simulink model "simQuadrotor"  (R2014b)
settings: Solver=ode45  StartTime=0.0  StopTime=tof  FixedStep=dt  MaxStep=dtmax  RelTol=1e-3
values from neighbouring files (symbols this model uses):
  a = (IzzT - IxxT)./ IxxT    [quadrotor.m]
  alpha = 1    [quadrotor.m]
  Aq = -20    [quadrotor.m]
  Ar = -10*eye(2)    [quadrotor.m]
  Arm = [-20 0 ; 0 -5]    [quadrotor.m]
  As = -50*eye(3)    [quadrotor.m]
  attitudeControlFlag = 4    [quadrotor.m]
  Bq = 1    [quadrotor.m]
  Br = [1 0]    [quadrotor.m]
  Dhat0 = zeros(3,1)    [quadrotor.m]
  Dlimit = 2.5    [quadrotor.m]
  DSecondLimit = 2    [quadrotor.m]
  dtFc = 10e-3    (= 0.01)    [quadrotor.m]
  epsilon = 0.1    [quadrotor.m]
  epsilontheta = 0.1    [quadrotor.m]
  euler0 = [0 0 0]'*pi/180    [quadrotor.m]
  Eulerc_ftc = [0 0 0]'    [quadrotor.m]
  faultyPropellerVec = double(not(faultyPropellerVec))    [quadrotor.m]
  FDstart = 3    [quadrotor.m]
  flims = [0.2*0 3.8*2.5]    [quadrotor.m]
  ftc_f2 = 0.1*2    (= 0.2)    [quadrotor.m]
  g = 9.81    [quadrotor.m]
  GammaW = 10000    [quadrotor.m]
  IxxB = IxxT - 4*IxxP    (= 0.0027)    [quadrotor.m]
  IxxT = 2.7e-3    (= 0.0027)    [quadrotor.m]
  IyyB = IyyT - 4*IyyP    (= 0.0027)    [quadrotor.m]
  IyyT = IxxT    (= 0.0027)    [quadrotor.m]
  IzzB = IzzT - 4*IzzP    (= 0.00514)    [quadrotor.m]
  IzzP = 1.5e-5    (= 1.5e-05)    [quadrotor.m]
  IzzT = 5.2e-3    (= 0.0052)    [quadrotor.m]
  Kdxx = 0.7e-4/10    (= 7e-06)    [quadrotor.m]
  Kdzz = 1.4e-4    (= 0.00014)    [quadrotor.m]
  Kf = 6.41e-6    (= 6.41e-06)    [quadrotor.m]
  Kp = 2*0.75*diag([1 1 1])    [quadrotor.m]
  Kp4 = 0.05    [quadrotor.m]
  Ktau = 1.72e-2    (= 0.0172)    [quadrotor.m]
  Kv = 0*0.005*diag([1 1 1])    [quadrotor.m]
  Kv4 = 0.02    [quadrotor.m]
  l = 0.17    [quadrotor.m]
  m = 0.5    [quadrotor.m]
  nc_ftc = 1    [quadrotor.m]
  nCheby = 3    [quadrotor.m]
  pqr0 = [0 0 0]'*pi/180    [quadrotor.m]
  Ps = lyap(As',Q)    [quadrotor.m]
  q0 = [euler0 ; pqr0]    [quadrotor.m]
  qp0 = 0    [quadrotor.m]
  sigmaMot = 0.015    [quadrotor.m]
  tfault = 5    [quadrotor.m]
  Vb0 = [0 0 0]'    [quadrotor.m]
  W0 = 0    [quadrotor.m]
  Wbnd = 10    [quadrotor.m]
  Xe0 = [0 0 0]'    [quadrotor.m]
  xhat0 = [pqr0]    [quadrotor.m]
undefined symbols (not defined in the file or in its folder): Intmax, Intmin, magnitude, rmax, rmin
libraries: aerolibutil x38, simulink x11, vrlib x3, dspbuff3 x1
(part 2 of 3)

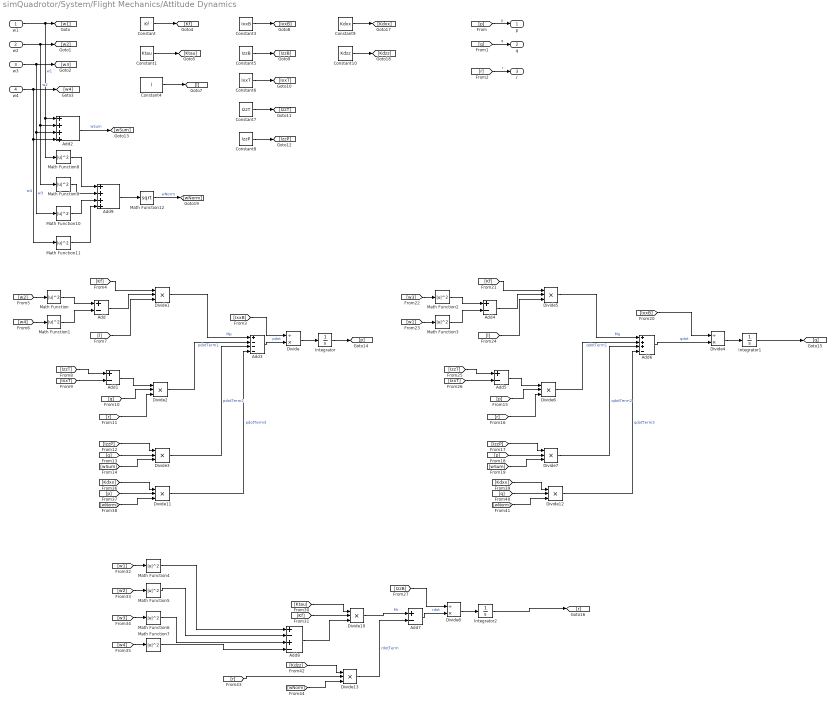
== system simQuadrotor/System/Flight Mechanics/Attitude Dynamics ==
  w1 : Inport
  w2 : Inport  Port=2
  w3 : Inport  Port=3
  w4 : Inport  Port=4
  Add{,1,4..5,7} (5 alike) : Sum  Inputs=+-
  Add2 : Sum  Inputs=++++
  Add3 : Sum  Inputs=+---
  Add6 : Sum  Inputs=+++-
  Add8 : Sum  Inputs=+-+-
  Add9 : Sum  Inputs=++++
  Constant : Constant  Value=Kf
  Constant1 : Constant  Value=Ktau
  Constant10 : Constant  Value=Kdzz
  Constant3 : Constant  Value=IxxB
  Constant4 : Constant  Value=l
  Constant5 : Constant  Value=IzzB
  Constant6 : Constant  Value=IxxT
  Constant7 : Constant  Value=IzzT
  Constant8 : Constant  Value=IzzP
  Constant9 : Constant  Value=Kdxx
  Divide : Product  Inputs=/*
  Divide{1..3,5..7,10..13} (10 alike) : Product  Inputs=***
  Divide4 : Product  Inputs=/*
  Divide8 : Product  Inputs=/*
  Integrator : Integrator  InitialCondition=pqr0(1)
  Integrator1 : Integrator  InitialCondition=pqr0(2)
  Integrator2 : Integrator  InitialCondition=pqr0(3)
  Math Function{,1..11} (12 alike) : Math  Operator=magnitude^2  SaturateOnIntegerOverflow=on
  Math Function12 : Math  Operator=sqrt  SaturateOnIntegerOverflow=on
  p : Outport
  q : Outport  Port=2
  r : Outport  Port=3
  wires:
  w1/1 -> [w1], Add2/1, Math Function8/1  "w1"
  w2/1 -> [w2], Add2/2, Math Function9/1  "w2"
  w3/1 -> [w3], Add2/3, Math Function10/1  "w3"
  w4/1 -> [w4], Add2/4, Math Function11/1  "w4"
  Constant4/1 -> [l]
  Constant1/1 -> [Ktau]
  Constant/1 -> [Kf]
  Constant3/1 -> [IxxB]
  Constant5/1 -> [IzzB]
  Constant6/1 -> [IxxT]
  Constant7/1 -> [IzzT]
  Constant8/1 -> [IzzP]
  [p] -> p/1  "p"
  [q] -> q/1  "q"
  [r] -> r/1  "r"
  Integrator/1 -> [p]
  Divide/1 -> Integrator/1
  [IxxB] -> Divide/1
  [Kf] -> Divide1/1
  [w2] -> Math Function/1
  [w4] -> Math Function1/1
  Math Function/1 -> Add/1
  Math Function1/1 -> Add/2
  Add/1 -> Divide1/2
  [l] -> Divide1/3
  [IzzT] -> Add1/1
  [IxxT] -> Add1/2
  Add1/1 -> Divide2/1
  [q] -> Divide2/2
  [r] -> Divide2/3
  Add2/1 -> [wSum]  "wSum"
  [IzzP] -> Divide3/1
  [q] -> Divide3/2
  [wSum] -> Divide3/3
  Add3/1 -> Divide/2  "pdot"
  Divide1/1 -> Add3/1  "Mp"
  Divide2/1 -> Add3/2  "pdotTerm1"
  Divide3/1 -> Add3/3  "pdotTerm2"
  Integrator1/1 -> [q]
  Divide4/1 -> Integrator1/1
  [IxxB] -> Divide4/1
  [Kf] -> Divide5/1
  [w3] -> Math Function2/1
  [w1] -> Math Function3/1
  Math Function2/1 -> Add4/1
  Math Function3/1 -> Add4/2
  Add4/1 -> Divide5/2
  [l] -> Divide5/3
  [IzzT] -> Add5/1
  [IxxT] -> Add5/2
  Add5/1 -> Divide6/1
  [p] -> Divide6/2
  [r] -> Divide6/3
  [IzzP] -> Divide7/1
  [p] -> Divide7/2
  [wSum] -> Divide7/3
  Add6/1 -> Divide4/2  "qdot"
  Divide5/1 -> Add6/1  "Mq"
  Divide6/1 -> Add6/2  "qdotTerm1"
  Divide7/1 -> Add6/3  "qdotTerm2"
  Integrator2/1 -> [r]
  Divide8/1 -> Integrator2/1
  [IzzB] -> Divide8/1
  Add7/1 -> Divide8/2  "rdot"
  [Ktau] -> Divide10/1
  [Kf] -> Divide10/2
  Add8/1 -> Divide10/3
  [w1] -> Math Function4/1
  [w2] -> Math Function5/1
  Math Function4/1 -> Add8/1
  Math Function5/1 -> Add8/2
  [w3] -> Math Function6/1
  [w4] -> Math Function7/1
  Math Function6/1 -> Add8/3
  Math Function7/1 -> Add8/4
  Constant9/1 -> [Kdxx]
  Constant10/1 -> [Kdzz]
  Math Function8/1 -> Add9/1
  Math Function9/1 -> Add9/2
  Math Function10/1 -> Add9/3
  Math Function11/1 -> Add9/4
  Add9/1 -> Math Function12/1
  Math Function12/1 -> [wNorm]  "wNorm"
  [Kdxx] -> Divide11/1
  [p] -> Divide11/2
  [wNorm] -> Divide11/3
  Divide11/1 -> Add3/4  "pdotTerm3"
  [Kdxx] -> Divide12/1
  [q] -> Divide12/2
  [wNorm] -> Divide12/3
  Divide12/1 -> Add6/4  "qdotTerm3"
  [Kdzz] -> Divide13/1
  [r] -> Divide13/2
  [wNorm] -> Divide13/3
  Divide10/1 -> Add7/1  "Mr"
  Divide13/1 -> Add7/2  "rdotTerm"

== system simQuadrotor/System/Flight Mechanics/DCM E to B ==
  phithetapsi : Inport
  Create 3x3 Matrix : aerolibutil/Create 3x3 Matrix
  Fcn11 : Fcn  Expr=u(5)*u(6)
  Fcn12 : Fcn  Expr=u(3)*u(5)
  Fcn13 : Fcn  Expr=-u(2)
  Fcn21 : Fcn  Expr=u(1)*u(2)*u(6)-u(4)*u(3)
  Fcn22 : Fcn  Expr=u(1)*u(2)*u(3)+u(4)*u(6)
  Fcn23 : Fcn  Expr=u(1)*u(5)
  Fcn31 : Fcn  Expr=u(4)*u(2)*u(6)+u(1)*u(3)
  Fcn32 : Fcn  Expr=u(4)*u(2)*u(3)-u(1)*u(6)
  Fcn33 : Fcn  Expr=u(4)*u(5)
  Mux : Mux  Inputs=2
  sincos : Trigonometry  Operator=sincos
  CB_E : Outport
  wires:
  sincos/1 -> Mux/1
  sincos/2 -> Mux/2
  Mux/1 -> Fcn32/1, Fcn33/1, Fcn31/1, Fcn23/1, Fcn22/1, Fcn11/1, Fcn12/1, Fcn13/1, Fcn21/1
  Fcn11/1 -> Create 3x3 Matrix/1
  Fcn12/1 -> Create 3x3 Matrix/2
  Fcn13/1 -> Create 3x3 Matrix/3
  Fcn21/1 -> Create 3x3 Matrix/4
  Fcn31/1 -> Create 3x3 Matrix/7
  Fcn22/1 -> Create 3x3 Matrix/5
  Fcn23/1 -> Create 3x3 Matrix/6
  Fcn32/1 -> Create 3x3 Matrix/8
  Fcn33/1 -> Create 3x3 Matrix/9
  phithetapsi/1 -> sincos/1  "phithetapsi"
  Create 3x3 Matrix/1 -> CB_E/1  "CB_E"

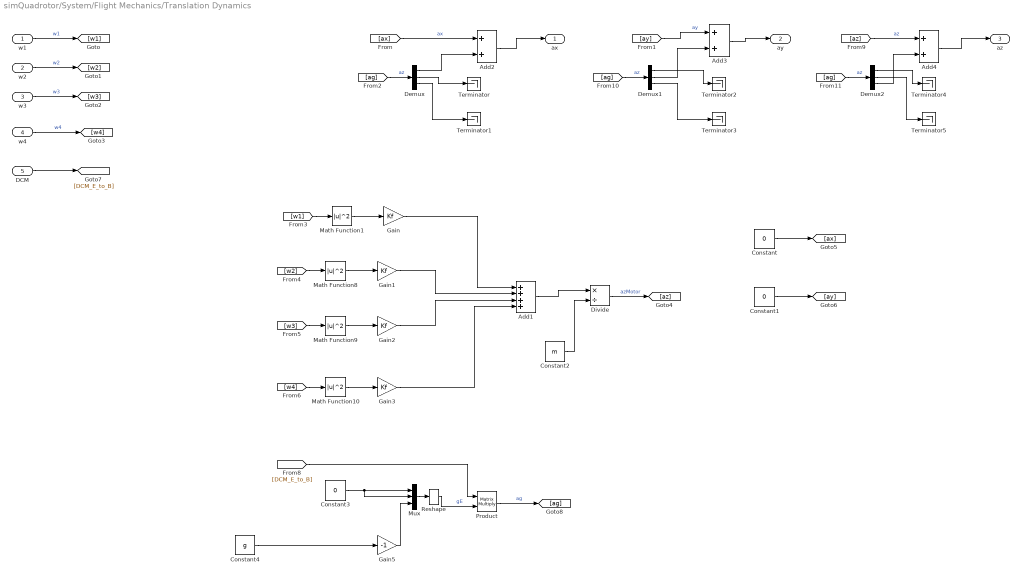
== system simQuadrotor/System/Flight Mechanics/Translation Dynamics ==
  w1 : Inport
  w2 : Inport  Port=2
  w3 : Inport  Port=3
  w4 : Inport  Port=4
  DCM : Inport  Port=5
  Add1 : Sum  Inputs=++++
  Add2 : Sum
  Add3 : Sum
  Add4 : Sum
  Constant : Constant  Value=0
  Constant1 : Constant  Value=0
  Constant2 : Constant  Value=m
  Constant3 : Constant  Value=0
  Constant4 : Constant  Value=g
  Demux : Demux  Outputs=3
  Demux1 : Demux  Outputs=3
  Demux2 : Demux  Outputs=3
  Divide : Product  Inputs=*/
  Gain{,1..3} (4 alike) : Gain  Gain=Kf
  Gain5 : Gain  Gain=-1
  Math Function{1,8..10} (4 alike) : Math  Operator=magnitude^2  SaturateOnIntegerOverflow=on
  Mux : Mux  Inputs=3
  Product : Product  Multiplication=Matrix(*)  RndMeth=Zero
  Reshape : Reshape  OutputDimensionality=Column vector (2-D)
  Terminator{,1..5} (6 alike) : Terminator
  ax : Outport
  ay : Outport  Port=2
  az : Outport  Port=3
  wires:
  w4/1 -> [w4]  "w4"
  w3/1 -> [w3]  "w3"
  w2/1 -> [w2]  "w2"
  w1/1 -> [w1]  "w1"
  [w1] -> Math Function1/1
  Math Function1/1 -> Gain/1
  [w2] -> Math Function8/1
  Math Function8/1 -> Gain1/1
  [w3] -> Math Function9/1
  Math Function9/1 -> Gain2/1
  [w4] -> Math Function10/1
  Math Function10/1 -> Gain3/1
  Gain/1 -> Add1/1
  Gain1/1 -> Add1/2
  Gain2/1 -> Add1/3
  Gain3/1 -> Add1/4
  Constant4/1 -> Gain5/1
  Constant/1 -> [ax]
  Constant1/1 -> [ay]
  Add1/1 -> Divide/1
  Divide/1 -> [az]  "azMotor"
  Constant2/1 -> Divide/2
  DCM/1 -> [DCM_E_to_B]
  [DCM_E_to_B] -> Product/1
  Constant3/1 -> Mux/1, Mux/2
  Gain5/1 -> Mux/3
  Mux/1 -> Reshape/1
  Reshape/1 -> Product/2  "gE"
  Product/1 -> [ag]  "ag"
  [ag] -> Demux/1  "az"
  [ax] -> Add2/1  "ax"
  Add2/1 -> ax/1
  [ay] -> Add3/1  "ay"
  Add3/1 -> ay/1
  [az] -> Add4/1  "az"
  Add4/1 -> az/1
  Demux/1 -> Add2/2
  [ag] -> Demux1/1  "az"
  Demux1/2 -> Add3/2
  [ag] -> Demux2/1  "az"
  Demux2/3 -> Add4/2
  Demux/2 -> Terminator/1
  Demux/3 -> Terminator1/1
  Demux1/1 -> Terminator2/1
  Demux1/3 -> Terminator3/1
  Demux2/1 -> Terminator4/1
  Demux2/2 -> Terminator5/1

== system simQuadrotor/System/Navigation/DCM E to B ==
  phithetapsi : Inport
  Create 3x3 Matrix : aerolibutil/Create 3x3 Matrix
  Fcn11 : Fcn  Expr=u(5)*u(6)
  Fcn12 : Fcn  Expr=u(3)*u(5)
  Fcn13 : Fcn  Expr=-u(2)
  Fcn21 : Fcn  Expr=u(1)*u(2)*u(6)-u(4)*u(3)
  Fcn22 : Fcn  Expr=u(1)*u(2)*u(3)+u(4)*u(6)
  Fcn23 : Fcn  Expr=u(1)*u(5)
  Fcn31 : Fcn  Expr=u(4)*u(2)*u(6)+u(1)*u(3)
  Fcn32 : Fcn  Expr=u(4)*u(2)*u(3)-u(1)*u(6)
  Fcn33 : Fcn  Expr=u(4)*u(5)
  Math Function : Math  Operator=transpose  SaturateOnIntegerOverflow=on
  Mux : Mux  Inputs=2
  Product : Product  Multiplication=Matrix(*)  RndMeth=Zero
  Product1 : Product  Inputs=/  Multiplication=Matrix(*)  RndMeth=Zero
  Terminator : Terminator
  Terminator1 : Terminator
  sincos : Trigonometry  Operator=sincos
  CB_E : Outport
  wires:
  sincos/1 -> Mux/1
  sincos/2 -> Mux/2
  Mux/1 -> Fcn32/1, Fcn33/1, Fcn31/1, Fcn23/1, Fcn22/1, Fcn11/1, Fcn12/1, Fcn13/1, Fcn21/1
  Fcn11/1 -> Create 3x3 Matrix/1
  Fcn12/1 -> Create 3x3 Matrix/2
  Fcn13/1 -> Create 3x3 Matrix/3
  Fcn21/1 -> Create 3x3 Matrix/4
  Fcn31/1 -> Create 3x3 Matrix/7
  Fcn22/1 -> Create 3x3 Matrix/5
  Fcn23/1 -> Create 3x3 Matrix/6
  Fcn32/1 -> Create 3x3 Matrix/8
  Fcn33/1 -> Create 3x3 Matrix/9
  phithetapsi/1 -> sincos/1  "phithetapsi"
  Create 3x3 Matrix/1 -> Math Function/1, CB_E/1, Product/1, Product1/1  "CB_E"
  Math Function/1 -> Product/2  "CB_ET"
  Product1/1 -> Terminator1/1  "CB_E_inv"
  Product/1 -> Terminator/1  "mult"

== system simQuadrotor/Controller/Disturbance Estimator/getDisturbance/Chebyshev Basis Functions ==
  x : Inport
  Chebyshev Polynomail Value Calculation : Subsystem  TreatAsAtomicUnit=on
  Demux : Demux  Outputs=3
  Mux : Mux  Inputs=3
  Reshape1 : Reshape  OutputDimensionality=Column vector (2-D)
  Reshape2 : Reshape  OutputDimensionality=Column vector (2-D)
  Tn : Outport
  wires:
  [Tn] -> Tn/1
  [z] -> Chebyshev Polynomail Value Calculation/1(x)
  Chebyshev Polynomail Value Calculation/1(chebyPol) -> Reshape2/1
  Reshape2/1 -> [Tn]
  x/1 -> [x]
  Mux/1 -> Reshape1/1
  Reshape1/1 -> [z]
  [x] -> Demux/1
  [wB2] -> Mux/2
  [wB3] -> Mux/3
  [wB1] -> Mux/1
  Demux/1 -> [wB1]
  Demux/2 -> [wB2]
  Demux/3 -> [wB3]

== system simQuadrotor/Controller/Disturbance Estimator/getDisturbance/getDhat ==
  psiz : Inport
  es : Inport  Port=2
  Bus Creator : BusCreator  Inputs=3
  Math Function : Math  Operator=transpose  SaturateOnIntegerOverflow=on
  Math Function1 : Math  Operator=transpose  SaturateOnIntegerOverflow=on
  Math Function2 : Math  Operator=transpose  SaturateOnIntegerOverflow=on
  Reshape : Reshape  OutputDimensionality=Column vector (2-D)
  Selector : Selector  NumberOfDimensions=2  InputPortWidth=3  IndexOptions=Select all,Index vector (dialog)  Indices=[1 3],1  OutputSizes=1,1
  Selector1 : Selector  NumberOfDimensions=2  InputPortWidth=3  IndexOptions=Select all,Index vector (dialog)  Indices=[1 3],2  OutputSizes=1,1
  Selector2 : Selector  NumberOfDimensions=2  InputPortWidth=3  IndexOptions=Select all,Index vector (dialog)  Indices=[1 3],3  OutputSizes=1,1
  Terminator1 : Terminator
  Vector Concatenate : Concatenate  NumInputs=3
  adaptiveGain : Subsystem  TreatAsAtomicUnit=on
  getW1 : Subsystem
  getW2 : Subsystem
  getW3 : Subsystem
  Dhat : Outport
  wires:
  es/1 -> [es]  "es"
  adaptiveGain/1(Wintegrand) -> [Wint]  "Wint"
  [Dhat] -> Dhat/1  "Dhat"
  psiz/1 -> [psiz]  "psiz"
  [es] -> adaptiveGain/2(es)
  [psiz] -> adaptiveGain/1(psi(z))
  [psiz] -> getW1/2(psiz)
  Selector/1 -> getW1/1(Wint)
  Vector Concatenate/1 -> Reshape/1
  [psiz] -> getW2/2(psiz)
  Selector1/1 -> getW2/1(Wint)
  Reshape/1 -> [Dhat]
  Bus Creator/1 -> Terminator1/1  "W"
  getW2/2(WTpsi) -> Vector Concatenate/2
  getW1/2(WTpsi) -> Vector Concatenate/1
  getW1/1(W) -> Math Function/1
  getW2/1(W) -> Math Function1/1
  [Wint] -> Selector2/1, Selector1/1, Selector/1
  Math Function/1 -> Bus Creator/1  "W1"
  Math Function1/1 -> Bus Creator/2  "W2"
  Selector2/1 -> getW3/1(Wint)
  [psiz] -> getW3/2(psiz)
  getW3/1(W) -> Math Function2/1
  Math Function2/1 -> Bus Creator/3
  getW3/2(WTpsi) -> Vector Concatenate/3  "W3"

== system simQuadrotor/Controller/FTC Controller/SingleProp Compensation/Motor Force Calculation ==
  fc : Inport
  u : Inport  Port=2
  Add2 : Sum  Inputs=+-
  Add3 : Sum
  Constant1 : Constant  Value=ftc_f2  VectorParams1D=off
  Constant3 : Constant  Value=0  VectorParams1D=off
  Gain1 : Gain  Gain=1/l
  Gain{3..4,9..10} (4 alike) : Gain  Gain=1/2
  Gain2 : Gain  Gain=1/l
  Mux : Mux
  Reshape : Reshape  OutputDimensionality=Column vector (2-D)
  fic : Outport
  wires:
  Gain4/1 -> Add3/1
  Gain3/1 -> Add2/1
  Gain2/1 -> Add3/2
  Gain1/1 -> Add2/2
  Gain10/1 -> Gain2/1
  Gain9/1 -> Gain1/1
  Constant1/1 -> [f2]
  u/1 -> [u]  "u"
  [f3] -> Mux/3
  [f1] -> Mux/1
  [f4] -> Mux/4
  [f2] -> Mux/2
  Constant3/1 -> [f4]
  Reshape/1 -> [fic]  "fic"
  Add3/1 -> [f3]
  [fc] -> Gain4/1
  [u] -> Gain10/1
  Add2/1 -> [f1]
  [fc] -> Gain3/1
  [u] -> Gain9/1
  Mux/1 -> Reshape/1
  [fic] -> fic/1
  fc/1 -> [fc]  "fc"

== system simQuadrotor/Controller/FTC Controller/SingleProp Compensation/PD-control for Reduced Attitude-Bullo ==
  r : Inport
  x : Inport  Port=2
  Add1 : Sum  Inputs=+-
  Constant1 : Constant  Value=0  VectorParams1D=off
  Gain4 : Gain  Gain=-1  Multiplication=Matrix(K*u)
  Gain5 : Gain  Gain=Kp4
  Gain6 : Gain  Gain=Kv4
  Math Function2 : Math  Operator=transpose  SaturateOnIntegerOverflow=on
  Math Function3 : Math  Operator=transpose  SaturateOnIntegerOverflow=on
  Mux : Mux  Inputs=2
  Mux1 : Mux  Inputs=2
  Mux2 : Mux  Inputs=2
  Product2 : Product  Multiplication=Matrix(*)  RndMeth=Zero
  Product3 : Product  Multiplication=Matrix(*)  RndMeth=Zero
  Product4 : Product  RndMeth=Zero
  Reshape{,1..4} (5 alike) : Reshape  OutputDimensionality=Column vector (2-D)
  "[4 5 6]" : Selector  InputPortWidth=6  Indices=4
  "[4 5 6]1" : Selector  InputPortWidth=6  Indices=5
  getRedAttRelatedPars : Subsystem
  Mc : Outport
  wires:
  Reshape4/1 -> [Mc]
  Constant1/1 -> Mux2/2
  Add1/1 -> Mux2/1
  Mux2/1 -> Reshape4/1
  Gain6/1 -> Add1/2  "Kvterm"
  Gain5/1 -> Add1/1  "Kpterm"
  Reshape2/1 -> Gain6/1
  [w2] -> Mux1/2
  [w1] -> Mux1/1
  Mux1/1 -> Reshape2/1
  Product4/1 -> Gain5/1
  Reshape/1 -> Product4/2
  [dist_pi0_q] -> Product4/1
  Mux/1 -> Reshape/1
  [V_Ypi1_V] -> Mux/2
  Gain4/1 -> Mux/1
  [V_Ypi2_V] -> Gain4/1
  [x] -> "[4 5 6]1"/1
  "[4 5 6]1"/1 -> Reshape1/1
  Reshape1/1 -> [w2]  "w2"
  [x] -> "[4 5 6]"/1
  "[4 5 6]"/1 -> Reshape3/1
  Reshape3/1 -> [w1]  "w1"
  Product3/1 -> [V_Ypi1_V]
  [pi1] -> Product3/2
  Math Function3/1 -> Product3/1
  [Yq_pi0] -> Math Function3/1
  Product2/1 -> [V_Ypi2_V]
  [pi2] -> Product2/2
  Math Function2/1 -> Product2/1
  [Yq_pi0] -> Math Function2/1
  getRedAttRelatedPars/4(pi2) -> [pi2]
  getRedAttRelatedPars/3(pi1) -> [pi1]
  getRedAttRelatedPars/1(Yq_pi0) -> [Yq_pi0]
  getRedAttRelatedPars/2(dist_pi0_q) -> [dist_pi0_q]
  [r] -> getRedAttRelatedPars/1(r)
  [x] -> getRedAttRelatedPars/2(x)
  [Mc] -> Mc/1  "Mc"
  x/1 -> [x]  "x"
  r/1 -> [r]  "r"

== system simQuadrotor/Controller/FTC Controller/SingleProp Compensation/Perturbation Calculation ==
  x : Inport
  qc : Inport  Port=2
  Add : Sum  Inputs=+-
  Add1 : Sum
  Add2 : Sum
  Add3 : Sum
  Constant1 : Constant  Value=Br  VectorParams1D=off
  Discrete-Time Integrator : DiscreteIntegrator  IntegratorMethod=Integration: Backward Euler  InitialCondition=qp0  InitialConditionSetting=State (most efficient)  SampleTime=-1  UpperSaturationLimit=rmax  LowerSaturationLimit=rmin
  Gain1 : Gain  Gain=Br'
  Gain2 : Gain  Gain=[0 0 0 0 1 0]'
  Gain3 : Gain  Gain=1/epsilon
  Gain4 : Gain  Gain=alpha
  Gain8 : Gain  Gain=Ar  Multiplication=Matrix(K*u)
  Memory3 : Memory  X0=qp0  InheritSampleTime=on  LinearizeMemory=on  LinearizeAsDelay=on
  Product1 : Product  Multiplication=Matrix(*)
  Reference model : Subsystem  TreatAsAtomicUnit=on
  Reshape2 : Reshape  OutputDimensionality=Column vector (2-D)
  System model : Subsystem  TreatAsAtomicUnit=on
  Terminator : Terminator
  getStates : Subsystem
  qp : Outport
  wires:
  [p2p] -> System model/5(p2p)
  [p1p] -> System model/4(p1p)
  getStates/5(p2p) -> [p2p]
  getStates/4(p1p) -> [p1p]
  [x2] -> Terminator/1
  Product1/1 -> [qp]
  [r] -> Product1/2
  Constant1/1 -> Product1/1
  [x1] -> System model/1(x1)
  getStates/3(w3) -> [w3]
  getStates/2(x2) -> [x2]
  getStates/1(x1) -> [x1]
  x/1 -> [x]  "x"
  [qp] -> qp/1
  System model/1(f1) -> [f1]  "f1"
  [w3] -> System model/2(w3)
  Reshape2/1 -> Memory3/1
  [r] -> Gain8/1
  Discrete-Time Integrator/1 -> Reshape2/1
  Gain3/1 -> Discrete-Time Integrator/1
  Memory3/1 -> [r]  "r"
  Gain8/1 -> Add2/2
  Reference model/1(f1r) -> [f1r]  "f1r"
  [x1] -> Reference model/1(x1)
  Add2/1 -> Gain3/1
  Gain4/1 -> Add2/1
  [f1r] -> Add/2
  [f1] -> Add/1
  Add/1 -> Gain4/1  "r_rhs"
  qc/1 -> [qc]  "qc"
  Add1/1 -> System model/3(r)
  [r] -> Add1/1
  [qc] -> Gain1/1
  Gain1/1 -> Add1/2
  [qc] -> Gain2/1
  [x] -> Add3/1
  Gain2/1 -> Add3/2
  Add3/1 -> getStates/1(x)

== system simQuadrotor/Controller/FTC Controller/SingleProp Compensation/Required Total Thrust ==
  x : Inport
  nc : Inport  Port=2
  Constant : Constant
  Constant1 : Constant  Value=m
  Constant2 : Constant  Value=g
  Product of Elements : Product  Inputs=*
  Product1 : Product  RndMeth=Zero
  Product2 : Product  Inputs=**/  RndMeth=Zero
  Selector : Selector  NumberOfDimensions=2  InputPortWidth=3  IndexOptions=Index vector (dialog),Index vector (dialog)  Indices=[1 2],1  OutputSizes=1,1
  Terminator : Terminator
  Trigonometric Function : Trigonometry  Operator=cos
  fc : Outport
  wires:
  Product1/1 -> Product2/2
  [nc] -> Product2/1
  nc/1 -> [nc]
  Trigonometric Function/1 -> Product of Elements/1
  Product of Elements/1 -> [cosphi_costht]
  Selector/1 -> Trigonometric Function/1
  Product2/1 -> fc/1
  Constant2/1 -> Product1/2
  Constant1/1 -> Product1/1
  x/1 -> Selector/1
  [cosphi_costht] -> Product2/3
  Constant/1 -> Terminator/1

== system simQuadrotor/Controller/FTC Controller/SingleProp Compensation/w3 Controller ==
  x : Inport
  qp : Inport  Port=2
  qc : Inport  Port=3
  Add1 : Sum
  Add2 : Sum  Inputs=++-
  Constant2 : Constant  Value=a  VectorParams1D=off
  Gain1 : Gain  Gain=Aq
  Gain2 : Gain  Gain=IyyT
  Gain3 : Gain  Gain=Bq
  Product1 : Product  Inputs=3  RndMeth=Zero
  Reshape1 : Reshape  OutputDimensionality=Column vector (2-D)
  Reshape3 : Reshape  OutputDimensionality=Column vector (2-D)
  Reshape5 : Reshape  OutputDimensionality=Column vector (2-D)
  "[4 5 6]" : Selector  InputPortWidth=6  Indices=4
  "[4 5 6]1" : Selector  InputPortWidth=6  Indices=6
  "[4 5 6]2" : Selector  InputPortWidth=6  Indices=5
  Mc : Outport
  wires:
  qp/1 -> [qp]  "qp"
  Gain2/1 -> [Mc]
  Add2/1 -> Gain2/1
  [w2] -> Gain1/1
  Reshape5/1 -> [w2]  "w2"
  "[4 5 6]2"/1 -> Reshape5/1
  [x] -> "[4 5 6]2"/1
  Constant2/1 -> Product1/1
  [w3] -> Product1/3
  [w1] -> Product1/2
  qc/1 -> [qc]  "qc"
  x/1 -> [x]  "x"
  [Mc] -> Mc/1  "Mc"
  Reshape3/1 -> [w1]  "w1"
  "[4 5 6]"/1 -> Reshape3/1
  [x] -> "[4 5 6]"/1
  Reshape1/1 -> [w3]  "w3"
  "[4 5 6]1"/1 -> Reshape1/1
  [x] -> "[4 5 6]1"/1
  Add1/1 -> Gain3/1  "qcommand"
  [qp] -> Add1/1
  [qc] -> Add1/2
  Gain3/1 -> Add2/1
  Gain1/1 -> Add2/2
  Product1/1 -> Add2/3

== system simQuadrotor/Controller/Nominal Controller/PD-Attitude Control with wB_IB/get eR ==
  r : Inport
  q : Inport  Port=2
  Add1 : Sum  Inputs=+-
  Add2 : Sum  Inputs=+-
  DCM E to B : Subsystem
  DCM E to B1 : Subsystem
  Product2 : Product  Inputs=/  Multiplication=Matrix(*)  RndMeth=Zero
  Product5 : Product  Inputs=/  Multiplication=Matrix(*)  RndMeth=Zero
  Product6 : Product  Multiplication=Matrix(*)  RndMeth=Zero
  Reshape{1..5} (5 alike) : Reshape  OutputDimensionality=Column vector (2-D)
  Terminator1 : Terminator
  Terminator2 : Terminator
  Terminator3 : Terminator
  "[ 1 2 3]" : Selector  NumberOfDimensions=2  InputPortWidth=3  IndexOptions=Index vector (dialog),Index vector (dialog)  Indices=[1 2 3],1  OutputSizes=1,1
  "[2 3 4]" : Selector  NumberOfDimensions=2  InputPortWidth=3  IndexOptions=Index vector (dialog),Index vector (dialog)  Indices=[2 3 4],1  OutputSizes=1,1
  "[4 5 6]" : Selector  NumberOfDimensions=2  InputPortWidth=3  IndexOptions=Index vector (dialog),Index vector (dialog)  Indices=[4 5 6],1  OutputSizes=1,1
  get Omega(R) RBAC : Subsystem
  get eR : Subsystem
  eR : Outport
  wires:
  [R] -> get eR/2(R)
  get eR/1(eR) -> [eR]  "eR"
  [Rc] -> get eR/1(Rc)
  [R] -> get Omega(R) RBAC/2(R)
  Product5/1 -> [R]
  Product2/1 -> [Rc]
  [q] -> Reshape5/1
  "[ 1 2 3]"/1 -> Reshape2/1
  "[4 5 6]"/1 -> Reshape3/1
  Reshape5/1 -> "[ 1 2 3]"/1, "[4 5 6]"/1
  [Rc] -> Product6/1  "RcTR"
  [wB] -> Product6/2
  [wB] -> Add1/1
  Product6/1 -> Add1/2  "RcTRpqr"
  Add1/1 -> Terminator1/1  "eM"
  [Euler] -> Add2/1
  [Eulerc] -> Add2/2
  Add2/1 -> Terminator2/1  "eEuler"
  get Omega(R) RBAC/1(Omega(R)) -> Terminator3/1  "Omega_R_"
  [Rc] -> get Omega(R) RBAC/1(Rc)
  Reshape1/1 -> [Eulerc]
  "[2 3 4]"/1 -> Reshape1/1
  [r] -> Reshape4/1
  Reshape2/1 -> [Euler]  "Euler"
  Reshape3/1 -> [wB]  "wB"
  Reshape4/1 -> "[2 3 4]"/1
  [Eulerc] -> DCM E to B/1(phithetapsi)
  DCM E to B/1(CB_E) -> Product2/1
  [Euler] -> DCM E to B1/1(phithetapsi)
  DCM E to B1/1(CB_E) -> Product5/1
  [eR] -> eR/1
  r/1 -> [r]  "r"
  q/1 -> [q]  "q"

== system simQuadrotor/Controller/Nominal Controller/PD-control for Attitude/DCM E to B ==
  phithetapsi : Inport
  Create 3x3 Matrix : aerolibutil/Create 3x3 Matrix
  Fcn11 : Fcn  Expr=u(5)*u(6)
  Fcn12 : Fcn  Expr=u(3)*u(5)
  Fcn13 : Fcn  Expr=-u(2)
  Fcn21 : Fcn  Expr=u(1)*u(2)*u(6)-u(4)*u(3)
  Fcn22 : Fcn  Expr=u(1)*u(2)*u(3)+u(4)*u(6)
  Fcn23 : Fcn  Expr=u(1)*u(5)
  Fcn31 : Fcn  Expr=u(4)*u(2)*u(6)+u(1)*u(3)
  Fcn32 : Fcn  Expr=u(4)*u(2)*u(3)-u(1)*u(6)
  Fcn33 : Fcn  Expr=u(4)*u(5)
  Mux : Mux  Inputs=2
  sincos : Trigonometry  Operator=sincos
  CB_E : Outport
  wires:
  Create 3x3 Matrix/1 -> CB_E/1  "CB_E"
  phithetapsi/1 -> sincos/1  "phithetapsi"
  Fcn33/1 -> Create 3x3 Matrix/9
  Fcn32/1 -> Create 3x3 Matrix/8
  Fcn23/1 -> Create 3x3 Matrix/6
  Fcn22/1 -> Create 3x3 Matrix/5
  Fcn31/1 -> Create 3x3 Matrix/7
  Fcn21/1 -> Create 3x3 Matrix/4
  Fcn13/1 -> Create 3x3 Matrix/3
  Fcn12/1 -> Create 3x3 Matrix/2
  Fcn11/1 -> Create 3x3 Matrix/1
  Mux/1 -> Fcn21/1, Fcn13/1, Fcn12/1, Fcn11/1, Fcn22/1, Fcn23/1, Fcn31/1, Fcn33/1, Fcn32/1
  sincos/2 -> Mux/2
  sincos/1 -> Mux/1

== system simQuadrotor/Controller/Nominal Controller/PD-control for Attitude/DCM E to B1 ==
  phithetapsi : Inport
  Create 3x3 Matrix : aerolibutil/Create 3x3 Matrix
  Fcn11 : Fcn  Expr=u(5)*u(6)
  Fcn12 : Fcn  Expr=u(3)*u(5)
  Fcn13 : Fcn  Expr=-u(2)
  Fcn21 : Fcn  Expr=u(1)*u(2)*u(6)-u(4)*u(3)
  Fcn22 : Fcn  Expr=u(1)*u(2)*u(3)+u(4)*u(6)
  Fcn23 : Fcn  Expr=u(1)*u(5)
  Fcn31 : Fcn  Expr=u(4)*u(2)*u(6)+u(1)*u(3)
  Fcn32 : Fcn  Expr=u(4)*u(2)*u(3)-u(1)*u(6)
  Fcn33 : Fcn  Expr=u(4)*u(5)
  Mux : Mux  Inputs=2
  sincos : Trigonometry  Operator=sincos
  CB_E : Outport
  wires:
  Create 3x3 Matrix/1 -> CB_E/1  "CB_E"
  phithetapsi/1 -> sincos/1  "phithetapsi"
  Fcn33/1 -> Create 3x3 Matrix/9
  Fcn32/1 -> Create 3x3 Matrix/8
  Fcn23/1 -> Create 3x3 Matrix/6
  Fcn22/1 -> Create 3x3 Matrix/5
  Fcn31/1 -> Create 3x3 Matrix/7
  Fcn21/1 -> Create 3x3 Matrix/4
  Fcn13/1 -> Create 3x3 Matrix/3
  Fcn12/1 -> Create 3x3 Matrix/2
  Fcn11/1 -> Create 3x3 Matrix/1
  Mux/1 -> Fcn21/1, Fcn13/1, Fcn12/1, Fcn11/1, Fcn22/1, Fcn23/1, Fcn31/1, Fcn33/1, Fcn32/1
  sincos/2 -> Mux/2
  sincos/1 -> Mux/1

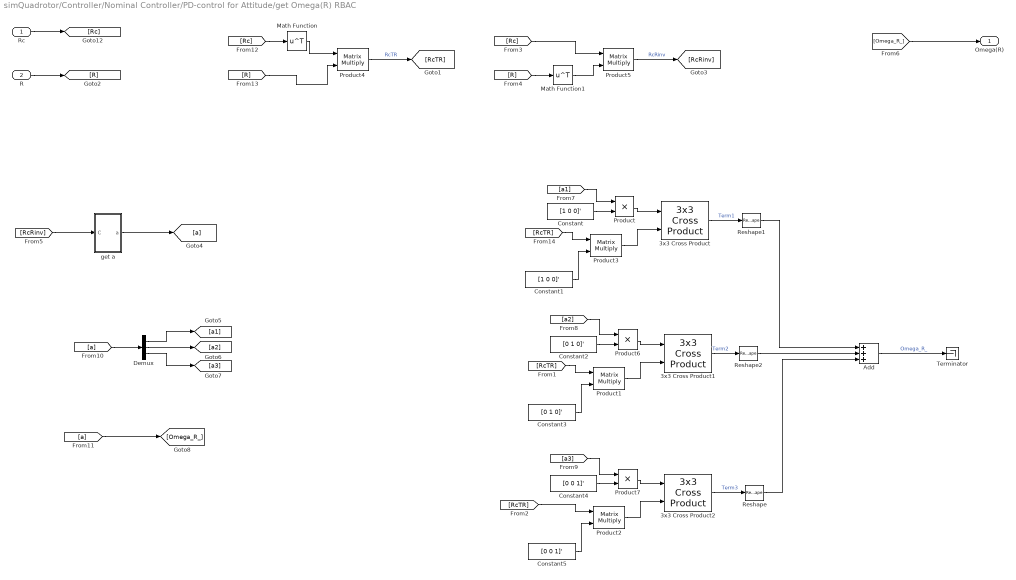
== system simQuadrotor/Controller/Nominal Controller/PD-control for Attitude/get Omega(R) RBAC ==
  Rc : Inport
  R : Inport  Port=2
  3x3 Cross Product : aerolibutil/3x3 Cross Product
  3x3 Cross Product1 : aerolibutil/3x3 Cross Product
  3x3 Cross Product2 : aerolibutil/3x3 Cross Product
  Add : Sum  Inputs=+++
  Constant : Constant  Value=[1 0 0]'  VectorParams1D=off
  Constant1 : Constant  Value=[1 0 0]'  VectorParams1D=off
  Constant2 : Constant  Value=[0 1 0]'  VectorParams1D=off
  Constant3 : Constant  Value=[0 1 0]'  VectorParams1D=off
  Constant4 : Constant  Value=[0 0 1]'  VectorParams1D=off
  Constant5 : Constant  Value=[0 0 1]'  VectorParams1D=off
  Demux : Demux  Outputs=3
  Math Function : Math  Operator=transpose  SaturateOnIntegerOverflow=on
  Math Function1 : Math  Operator=transpose  SaturateOnIntegerOverflow=on
  Product : Product  RndMeth=Zero
  Product{1..5} (5 alike) : Product  Multiplication=Matrix(*)  RndMeth=Zero
  Product6 : Product  RndMeth=Zero
  Product7 : Product  RndMeth=Zero
  Reshape : Reshape  OutputDimensionality=Column vector (2-D)
  Reshape1 : Reshape  OutputDimensionality=Column vector (2-D)
  Reshape2 : Reshape  OutputDimensionality=Column vector (2-D)
  Terminator : Terminator
  get a : Subsystem
  Omega(R) : Outport
  wires:
  [a] -> [Omega_R_]
  Reshape/1 -> Add/3
  Reshape2/1 -> Add/2
  Reshape1/1 -> Add/1
  Demux/3 -> [a3]
  Demux/2 -> [a2]
  Demux/1 -> [a1]
  [a] -> Demux/1
  [a3] -> Product7/1
  [a2] -> Product6/1
  [a1] -> Product/1
  get a/1(a) -> [a]
  [RcRinv] -> get a/1(C)
  Math Function1/1 -> Product5/2
  Product5/1 -> [RcRinv]  "RcRinv"
  [R] -> Math Function1/1
  [Rc] -> Product5/1
  R/1 -> [R]
  Rc/1 -> [Rc]
  Math Function/1 -> Product4/1
  Product4/1 -> [RcTR]  "RcTR"
  [R] -> Product4/2
  [Rc] -> Math Function/1
  [Omega_R_] -> Omega(R)/1
  Add/1 -> Terminator/1  "Omega_R_"
  3x3 Cross Product2/1 -> Reshape/1  "Term3"
  3x3 Cross Product1/1 -> Reshape2/1  "Term2"
  3x3 Cross Product/1 -> Reshape1/1  "Term1"
  Product7/1 -> 3x3 Cross Product2/1
  Product2/1 -> 3x3 Cross Product2/2
  Constant5/1 -> Product2/2
  [RcTR] -> Product2/1
  Constant4/1 -> Product7/2
  Product6/1 -> 3x3 Cross Product1/1
  Product/1 -> 3x3 Cross Product/1
  Product1/1 -> 3x3 Cross Product1/2
  Constant3/1 -> Product1/2
  [RcTR] -> Product1/1
  Constant2/1 -> Product6/2
  Product3/1 -> 3x3 Cross Product/2
  Constant1/1 -> Product3/2
  [RcTR] -> Product3/1
  Constant/1 -> Product/2

== system simQuadrotor/Controller/Nominal Controller/PD-control for Attitude/get eR ==
  note: Vee map
  Rc : Inport
  R : Inport  Port=2
  13 : Selector  NumberOfDimensions=2  InputPortWidth=3  IndexOptions=Index vector (dialog),Index vector (dialog)  Indices=1,3  OutputSizes=1,1
  21 : Selector  NumberOfDimensions=2  InputPortWidth=3  IndexOptions=Index vector (dialog),Index vector (dialog)  Indices=2,1  OutputSizes=1,1
  32 : Selector  NumberOfDimensions=2  InputPortWidth=3  IndexOptions=Index vector (dialog),Index vector (dialog)  Indices=3,2  OutputSizes=1,1
  Add : Sum  Inputs=+-
  Gain4 : Gain  Gain=1/2
  Math Function1 : Math  Operator=transpose  SaturateOnIntegerOverflow=on
  Math Function2 : Math  Operator=transpose  SaturateOnIntegerOverflow=on
  Math Function3 : Math  Operator=transpose  SaturateOnIntegerOverflow=on
  Mux : Mux  Inputs=3
  Product : Product  RndMeth=Zero
  Product1 : Product  Multiplication=Matrix(*)  RndMeth=Zero
  Product2 : Product  Multiplication=Matrix(*)  RndMeth=Zero
  Product5 : Product  Multiplication=Matrix(*)  RndMeth=Zero
  Reshape6 : Reshape  OutputDimensionality=Column vector (2-D)
  get alpha : Subsystem
  eR : Outport
  wires:
  Product/1 -> [eR]
  [alpha] -> Product/2
  Reshape6/1 -> Product/1  "eR_non"
  [Rc] -> Math Function2/1
  Math Function2/1 -> Product1/1
  [R] -> Product1/2
  [R] -> Math Function3/1
  Math Function3/1 -> Product2/1
  [Rc] -> Product2/2
  Product1/1 -> Add/1  "RcTR"
  Product2/1 -> Add/2  "RTRc"
  Add/1 -> Gain4/1
  Gain4/1 -> 32/1, 21/1, 13/1
  32/1 -> Mux/1
  13/1 -> Mux/2
  21/1 -> Mux/3
  Mux/1 -> Reshape6/1
  [RcRinv] -> get alpha/1(C)
  get alpha/1(alpha) -> [alpha]  "alpha"
  [eR] -> eR/1
  Rc/1 -> [Rc]
  R/1 -> [R]
  [Rc] -> Product5/1
  [R] -> Math Function1/1
  Product5/1 -> [RcRinv]  "RcRinv"
  Math Function1/1 -> Product5/2

== system simQuadrotor/Controller/Nominal Controller/PD-control for AttitudeAlt/DCM E to B ==
  phithetapsi : Inport
  Create 3x3 Matrix : aerolibutil/Create 3x3 Matrix
  Fcn11 : Fcn  Expr=u(5)*u(6)
  Fcn12 : Fcn  Expr=u(3)*u(5)
  Fcn13 : Fcn  Expr=-u(2)
  Fcn21 : Fcn  Expr=u(1)*u(2)*u(6)-u(4)*u(3)
  Fcn22 : Fcn  Expr=u(1)*u(2)*u(3)+u(4)*u(6)
  Fcn23 : Fcn  Expr=u(1)*u(5)
  Fcn31 : Fcn  Expr=u(4)*u(2)*u(6)+u(1)*u(3)
  Fcn32 : Fcn  Expr=u(4)*u(2)*u(3)-u(1)*u(6)
  Fcn33 : Fcn  Expr=u(4)*u(5)
  Mux : Mux  Inputs=2
  sincos : Trigonometry  Operator=sincos
  CB_E : Outport
  wires:
  sincos/1 -> Mux/1
  sincos/2 -> Mux/2
  Mux/1 -> Fcn32/1, Fcn33/1, Fcn31/1, Fcn23/1, Fcn22/1, Fcn11/1, Fcn12/1, Fcn13/1, Fcn21/1
  Fcn11/1 -> Create 3x3 Matrix/1
  Fcn12/1 -> Create 3x3 Matrix/2
  Fcn13/1 -> Create 3x3 Matrix/3
  Fcn21/1 -> Create 3x3 Matrix/4
  Fcn31/1 -> Create 3x3 Matrix/7
  Fcn22/1 -> Create 3x3 Matrix/5
  Fcn23/1 -> Create 3x3 Matrix/6
  Fcn32/1 -> Create 3x3 Matrix/8
  Fcn33/1 -> Create 3x3 Matrix/9
  phithetapsi/1 -> sincos/1  "phithetapsi"
  Create 3x3 Matrix/1 -> CB_E/1  "CB_E"

== system simQuadrotor/Controller/Nominal Controller/PD-control for AttitudeAlt/DCM E to B1 ==
  phithetapsi : Inport
  Create 3x3 Matrix : aerolibutil/Create 3x3 Matrix
  Fcn11 : Fcn  Expr=u(5)*u(6)
  Fcn12 : Fcn  Expr=u(3)*u(5)
  Fcn13 : Fcn  Expr=-u(2)
  Fcn21 : Fcn  Expr=u(1)*u(2)*u(6)-u(4)*u(3)
  Fcn22 : Fcn  Expr=u(1)*u(2)*u(3)+u(4)*u(6)
  Fcn23 : Fcn  Expr=u(1)*u(5)
  Fcn31 : Fcn  Expr=u(4)*u(2)*u(6)+u(1)*u(3)
  Fcn32 : Fcn  Expr=u(4)*u(2)*u(3)-u(1)*u(6)
  Fcn33 : Fcn  Expr=u(4)*u(5)
  Mux : Mux  Inputs=2
  sincos : Trigonometry  Operator=sincos
  CB_E : Outport
  wires:
  sincos/1 -> Mux/1
  sincos/2 -> Mux/2
  Mux/1 -> Fcn32/1, Fcn33/1, Fcn31/1, Fcn23/1, Fcn22/1, Fcn11/1, Fcn12/1, Fcn13/1, Fcn21/1
  Fcn11/1 -> Create 3x3 Matrix/1
  Fcn12/1 -> Create 3x3 Matrix/2
  Fcn13/1 -> Create 3x3 Matrix/3
  Fcn21/1 -> Create 3x3 Matrix/4
  Fcn31/1 -> Create 3x3 Matrix/7
  Fcn22/1 -> Create 3x3 Matrix/5
  Fcn23/1 -> Create 3x3 Matrix/6
  Fcn32/1 -> Create 3x3 Matrix/8
  Fcn33/1 -> Create 3x3 Matrix/9
  phithetapsi/1 -> sincos/1  "phithetapsi"
  Create 3x3 Matrix/1 -> CB_E/1  "CB_E"

== system simQuadrotor/Controller/Nominal Controller/PD-control for AttitudeAlt/get Omega(R) RBAC ==
  Rc : Inport
  R : Inport  Port=2
  3x3 Cross Product : aerolibutil/3x3 Cross Product
  3x3 Cross Product1 : aerolibutil/3x3 Cross Product
  3x3 Cross Product2 : aerolibutil/3x3 Cross Product
  Add : Sum  Inputs=+++
  Constant : Constant  Value=[1 0 0]'  VectorParams1D=off
  Constant1 : Constant  Value=[1 0 0]'  VectorParams1D=off
  Constant2 : Constant  Value=[0 1 0]'  VectorParams1D=off
  Constant3 : Constant  Value=[0 1 0]'  VectorParams1D=off
  Constant4 : Constant  Value=[0 0 1]'  VectorParams1D=off
  Constant5 : Constant  Value=[0 0 1]'  VectorParams1D=off
  Demux : Demux  Outputs=3
  Ground : Ground
  Math Function : Math  Operator=transpose  SaturateOnIntegerOverflow=on
  Product : Product  RndMeth=Zero
  Product{1..4} (4 alike) : Product  Multiplication=Matrix(*)  RndMeth=Zero
  Product6 : Product  RndMeth=Zero
  Product7 : Product  RndMeth=Zero
  Reshape : Reshape  OutputDimensionality=Column vector (2-D)
  Reshape1 : Reshape  OutputDimensionality=Column vector (2-D)
  Reshape2 : Reshape  OutputDimensionality=Column vector (2-D)
  Terminator1 : Terminator
  get a : Subsystem
  get a1_old : Subsystem
  Omega(R) : Outport
  wires:
  Constant/1 -> Product/2
  [RcTR] -> Product3/1
  Constant1/1 -> Product3/2
  Product3/1 -> 3x3 Cross Product/2
  Constant2/1 -> Product6/2
  [RcTR] -> Product1/1
  Constant3/1 -> Product1/2
  Product1/1 -> 3x3 Cross Product1/2
  Product/1 -> 3x3 Cross Product/1
  Product6/1 -> 3x3 Cross Product1/1
  Constant4/1 -> Product7/2
  [RcTR] -> Product2/1
  Constant5/1 -> Product2/2
  Product2/1 -> 3x3 Cross Product2/2
  Product7/1 -> 3x3 Cross Product2/1
  3x3 Cross Product/1 -> Reshape1/1  "Term1"
  3x3 Cross Product1/1 -> Reshape2/1  "Term2"
  3x3 Cross Product2/1 -> Reshape/1  "Term3"
  Add/1 -> [Omega_R_]  "Omega_R_"
  [Omega_R_] -> Omega(R)/1
  [Rc] -> Math Function/1
  [R] -> Product4/2
  Product4/1 -> [RcTR]  "RcTR"
  Math Function/1 -> Product4/1
  Rc/1 -> [Rc]
  R/1 -> [R]
  get a/1(a) -> [a]
  [a1] -> Product/1
  [a2] -> Product6/1
  [a3] -> Product7/1
  [a] -> Demux/1
  Demux/1 -> [a1]
  Demux/2 -> [a2]
  Demux/3 -> [a3]
  Reshape1/1 -> Add/1
  Reshape2/1 -> Add/2
  Reshape/1 -> Add/3
  get a1_old/1(a) -> Terminator1/1
  Ground/1 -> get a1_old/1(C)
  [Rc] -> get a/2(Rc)
  [R] -> get a/1(R)

== system simQuadrotor/Controller/Nominal Controller/PD-control for AttitudeAlt/get eR ==
  note: Vee map
  Rc : Inport
  R : Inport  Port=2
  13 : Selector  NumberOfDimensions=2  InputPortWidth=3  IndexOptions=Index vector (dialog),Index vector (dialog)  Indices=1,3  OutputSizes=1,1
  21 : Selector  NumberOfDimensions=2  InputPortWidth=3  IndexOptions=Index vector (dialog),Index vector (dialog)  Indices=2,1  OutputSizes=1,1
  32 : Selector  NumberOfDimensions=2  InputPortWidth=3  IndexOptions=Index vector (dialog),Index vector (dialog)  Indices=3,2  OutputSizes=1,1
  Add : Sum  Inputs=+-
  Gain4 : Gain  Gain=1/2
  Math Function1 : Math  Operator=transpose  SaturateOnIntegerOverflow=on
  Math Function2 : Math  Operator=transpose  SaturateOnIntegerOverflow=on
  Math Function3 : Math  Operator=transpose  SaturateOnIntegerOverflow=on
  Mux : Mux  Inputs=3
  Product : Product  RndMeth=Zero
  Product1 : Product  Multiplication=Matrix(*)  RndMeth=Zero
  Product2 : Product  Multiplication=Matrix(*)  RndMeth=Zero
  Product5 : Product  Multiplication=Matrix(*)  RndMeth=Zero
  Reshape6 : Reshape  OutputDimensionality=Column vector (2-D)
  get alpha : Subsystem
  eR : Outport
  wires:
  Math Function1/1 -> Product5/2
  Product5/1 -> [RcRinv]  "RcRinv"
  [R] -> Math Function1/1
  [Rc] -> Product5/1
  R/1 -> [R]
  Rc/1 -> [Rc]
  [eR] -> eR/1
  get alpha/1(alpha) -> [alpha]  "alpha"
  [RcRinv] -> get alpha/1(C)
  Mux/1 -> Reshape6/1
  21/1 -> Mux/3
  13/1 -> Mux/2
  32/1 -> Mux/1
  Gain4/1 -> 13/1, 21/1, 32/1
  Add/1 -> Gain4/1
  Product2/1 -> Add/2  "RTRc"
  Product1/1 -> Add/1  "RcTR"
  [Rc] -> Product2/2
  Math Function3/1 -> Product2/1
  [R] -> Math Function3/1
  [R] -> Product1/2
  Math Function2/1 -> Product1/1
  [Rc] -> Math Function2/1
  Reshape6/1 -> Product/1  "eR_non"
  [alpha] -> Product/2
  Product/1 -> [eR]

== system simQuadrotor/Controller/Nominal Controller/PD-control for Reduced Attitude/DCM E to B ==
  phithetapsi : Inport
  Create 3x3 Matrix : aerolibutil/Create 3x3 Matrix
  Fcn11 : Fcn  Expr=u(5)*u(6)
  Fcn12 : Fcn  Expr=u(3)*u(5)
  Fcn13 : Fcn  Expr=-u(2)
  Fcn21 : Fcn  Expr=u(1)*u(2)*u(6)-u(4)*u(3)
  Fcn22 : Fcn  Expr=u(1)*u(2)*u(3)+u(4)*u(6)
  Fcn23 : Fcn  Expr=u(1)*u(5)
  Fcn31 : Fcn  Expr=u(4)*u(2)*u(6)+u(1)*u(3)
  Fcn32 : Fcn  Expr=u(4)*u(2)*u(3)-u(1)*u(6)
  Fcn33 : Fcn  Expr=u(4)*u(5)
  Mux : Mux  Inputs=2
  sincos : Trigonometry  Operator=sincos
  CB_E : Outport
  wires:
  Create 3x3 Matrix/1 -> CB_E/1  "CB_E"
  phithetapsi/1 -> sincos/1  "phithetapsi"
  Fcn33/1 -> Create 3x3 Matrix/9
  Fcn32/1 -> Create 3x3 Matrix/8
  Fcn23/1 -> Create 3x3 Matrix/6
  Fcn22/1 -> Create 3x3 Matrix/5
  Fcn31/1 -> Create 3x3 Matrix/7
  Fcn21/1 -> Create 3x3 Matrix/4
  Fcn13/1 -> Create 3x3 Matrix/3
  Fcn12/1 -> Create 3x3 Matrix/2
  Fcn11/1 -> Create 3x3 Matrix/1
  Mux/1 -> Fcn21/1, Fcn13/1, Fcn12/1, Fcn11/1, Fcn22/1, Fcn23/1, Fcn31/1, Fcn33/1, Fcn32/1
  sincos/2 -> Mux/2
  sincos/1 -> Mux/1

== system simQuadrotor/Controller/Nominal Controller/PD-control for Reduced Attitude/DCM E to B1 ==
  phithetapsi : Inport
  Create 3x3 Matrix : aerolibutil/Create 3x3 Matrix
  Fcn11 : Fcn  Expr=u(5)*u(6)
  Fcn12 : Fcn  Expr=u(3)*u(5)
  Fcn13 : Fcn  Expr=-u(2)
  Fcn21 : Fcn  Expr=u(1)*u(2)*u(6)-u(4)*u(3)
  Fcn22 : Fcn  Expr=u(1)*u(2)*u(3)+u(4)*u(6)
  Fcn23 : Fcn  Expr=u(1)*u(5)
  Fcn31 : Fcn  Expr=u(4)*u(2)*u(6)+u(1)*u(3)
  Fcn32 : Fcn  Expr=u(4)*u(2)*u(3)-u(1)*u(6)
  Fcn33 : Fcn  Expr=u(4)*u(5)
  Mux : Mux  Inputs=2
  sincos : Trigonometry  Operator=sincos
  CB_E : Outport
  wires:
  Create 3x3 Matrix/1 -> CB_E/1  "CB_E"
  phithetapsi/1 -> sincos/1  "phithetapsi"
  Fcn33/1 -> Create 3x3 Matrix/9
  Fcn32/1 -> Create 3x3 Matrix/8
  Fcn23/1 -> Create 3x3 Matrix/6
  Fcn22/1 -> Create 3x3 Matrix/5
  Fcn31/1 -> Create 3x3 Matrix/7
  Fcn21/1 -> Create 3x3 Matrix/4
  Fcn13/1 -> Create 3x3 Matrix/3
  Fcn12/1 -> Create 3x3 Matrix/2
  Fcn11/1 -> Create 3x3 Matrix/1
  Mux/1 -> Fcn21/1, Fcn13/1, Fcn12/1, Fcn11/1, Fcn22/1, Fcn23/1, Fcn31/1, Fcn33/1, Fcn32/1
  sincos/2 -> Mux/2
  sincos/1 -> Mux/1

== system simQuadrotor/Controller/Nominal Controller/PD-control for Reduced Attitude/get alpha ==
  C : Inport
  11 : Selector  NumberOfDimensions=2  InputPortWidth=3  IndexOptions=Index vector (dialog),Index vector (dialog)  Indices=1,1  OutputSizes=1,1
  22 : Selector  NumberOfDimensions=2  InputPortWidth=3  IndexOptions=Index vector (dialog),Index vector (dialog)  Indices=2,2  OutputSizes=1,1
  33 : Selector  NumberOfDimensions=2  InputPortWidth=3  IndexOptions=Index vector (dialog),Index vector (dialog)  Indices=3,3  OutputSizes=1,1
  Add : Sum  Inputs=+++-
  Constant5 : Constant
  Gain1 : Gain  Gain=0.5
  Trigonometric Function : Trigonometry  Operator=acos
  alpha : Outport
  wires:
  C/1 -> 33/1, 11/1, 22/1
  11/1 -> [C11]
  22/1 -> [C22]
  33/1 -> [C33]
  [C11] -> Add/1
  [C22] -> Add/2
  [C33] -> Add/3
  Constant5/1 -> Add/4
  Add/1 -> Gain1/1
  Gain1/1 -> Trigonometric Function/1
  Trigonometric Function/1 -> [alpha]  "alpha"
  [alpha] -> alpha/1

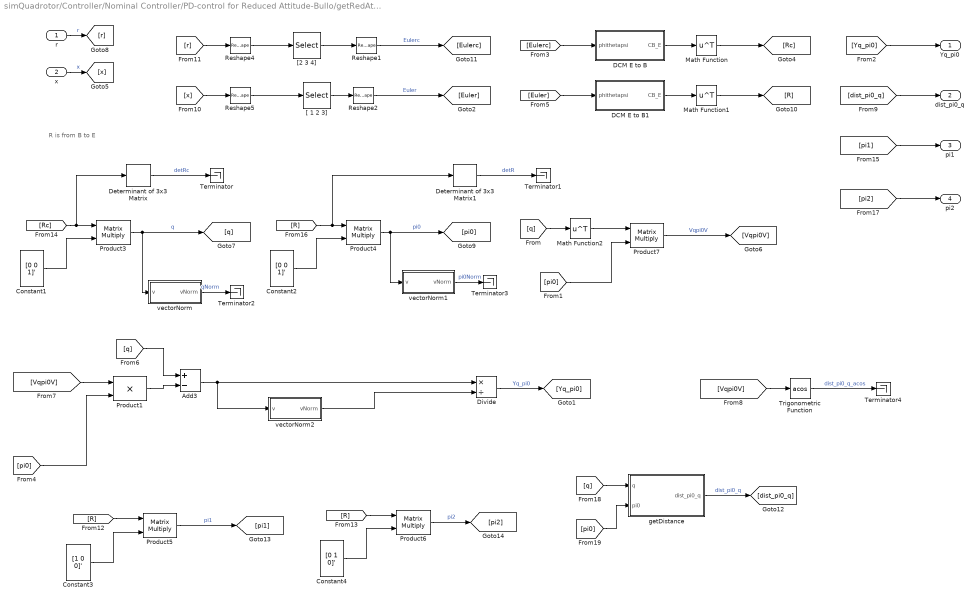
== system simQuadrotor/Controller/Nominal Controller/PD-control for Reduced Attitude-Bullo/getRedAttRelatedPars ==
  note: R is from B to E
  r : Inport
  x : Inport  Port=2
  Add3 : Sum  Inputs=+-
  Constant1 : Constant  Value=[0 0 1]'  VectorParams1D=off
  Constant2 : Constant  Value=[0 0 1]'  VectorParams1D=off
  Constant3 : Constant  Value=[1 0 0]'  VectorParams1D=off
  Constant4 : Constant  Value=[0 1 0]'  VectorParams1D=off
  DCM E to B : Subsystem
  DCM E to B1 : Subsystem
  Determinant of 3x3 Matrix : aerolibutil/Determinant of 3x3 Matrix
  Determinant of 3x3 Matrix1 : aerolibutil/Determinant of 3x3 Matrix
  Divide : Product  Inputs=*/
  Math Function : Math  Operator=transpose  SaturateOnIntegerOverflow=on
  Math Function1 : Math  Operator=transpose  SaturateOnIntegerOverflow=on
  Math Function2 : Math  Operator=transpose  SaturateOnIntegerOverflow=on
  Product1 : Product  RndMeth=Zero
  Product{3..7} (5 alike) : Product  Multiplication=Matrix(*)  RndMeth=Zero
  Reshape{1..2,4..5} (4 alike) : Reshape  OutputDimensionality=Column vector (2-D)
  Terminator{,1..4} (5 alike) : Terminator
  Trigonometric Function : Trigonometry  Operator=acos
  "[ 1 2 3]" : Selector  NumberOfDimensions=2  InputPortWidth=3  IndexOptions=Index vector (dialog),Index vector (dialog)  Indices=[1 2 3],1  OutputSizes=1,1
  "[2 3 4]" : Selector  NumberOfDimensions=2  InputPortWidth=3  IndexOptions=Index vector (dialog),Index vector (dialog)  Indices=[2 3 4],1  OutputSizes=1,1
  getDistance : Subsystem
  vectorNorm : Subsystem
  vectorNorm1 : Subsystem
  vectorNorm2 : Subsystem
  Yq_pi0 : Outport
  dist_pi0_q : Outport  Port=2
  pi1 : Outport  Port=3
  pi2 : Outport  Port=4
  wires:
  DCM E to B1/1(CB_E) -> Math Function1/1
  [Euler] -> DCM E to B1/1(phithetapsi)
  Reshape4/1 -> "[2 3 4]"/1
  DCM E to B/1(CB_E) -> Math Function/1
  [Eulerc] -> DCM E to B/1(phithetapsi)
  [r] -> Reshape4/1
  "[2 3 4]"/1 -> Reshape1/1
  Reshape1/1 -> [Eulerc]  "Eulerc"
  Reshape2/1 -> [Euler]  "Euler"
  Reshape5/1 -> "[ 1 2 3]"/1
  "[ 1 2 3]"/1 -> Reshape2/1
  Math Function/1 -> [Rc]
  [x] -> Reshape5/1
  Math Function1/1 -> [R]
  x/1 -> [x]  "x"
  r/1 -> [r]  "r"
  Product4/1 -> vectorNorm1/1(v), [pi0]  "pi0"
  Constant2/1 -> Product4/2
  [R] -> Determinant of 3x3 Matrix1/1, Product4/1
  Product3/1 -> vectorNorm/1(v), [q]  "q"
  Constant1/1 -> Product3/2
  [Rc] -> Determinant of 3x3 Matrix/1, Product3/1
  [dist_pi0_q] -> dist_pi0_q/1
  [q] -> Math Function2/1
  Math Function2/1 -> Product7/1
  [pi0] -> Product7/2
  [pi0] -> Product1/2
  [q] -> Add3/1
  Product1/1 -> Add3/2
  Add3/1 -> vectorNorm2/1(v), Divide/1
  vectorNorm2/1(vNorm) -> Divide/2
  Divide/1 -> [Yq_pi0]  "Yq_pi0"
  Product7/1 -> [Vqpi0V]  "Vqpi0V"
  [Vqpi0V] -> Product1/1
  [Vqpi0V] -> Trigonometric Function/1
  Trigonometric Function/1 -> Terminator4/1  "dist_pi0_q_acos"
  [Yq_pi0] -> Yq_pi0/1
  Product5/1 -> [pi1]  "pi1"
  Constant3/1 -> Product5/2
  [R] -> Product5/1
  Product6/1 -> [pi2]  "pi2"
  Constant4/1 -> Product6/2
  [R] -> Product6/1
  [pi1] -> pi1/1
  [pi2] -> pi2/1
  Determinant of 3x3 Matrix/1 -> Terminator/1  "detRc"
  Determinant of 3x3 Matrix1/1 -> Terminator1/1  "detR"
  vectorNorm/1(vNorm) -> Terminator2/1  "qNorm"
  vectorNorm1/1(vNorm) -> Terminator3/1  "pi0Norm"
  getDistance/1(dist_pi0_q) -> [dist_pi0_q]  "dist_pi0_q"
  [q] -> getDistance/1(q)
  [pi0] -> getDistance/2(pi0)

== system simQuadrotor/Controller/Disturbance Estimator/getDisturbance/Chebyshev Basis Functions/Chebyshev Polynomail Value Calculation ==
  x : Inport
  Delay Line : dspbuff3/Delay Line  siz=nCheby  ic=zeros(nCheby,1)  directfeed=on  enable_output=off  hold_output=off  TreatMby1Signals=M channels (this choice will be removed - see release notes)
  For Iterator : ForIterator  IterationLimit=nCheby
  Frame Conversion : FrameConversion  OutFrame=Sample-based
  If : If  IfExpression=u1 > 2
  If Action Subsystem : Subsystem  TreatAsAtomicUnit=on
  If Action Subsystem1 : Subsystem  TreatAsAtomicUnit=on
  Memory : Memory  InheritSampleTime=on  LinearizeMemory=on  LinearizeAsDelay=on
  Merge : Merge
  Reshape : Reshape  OutputDimensionality=Column vector (2-D)
  chebyPol : Outport
  wires:
  For Iterator/1 -> [N]
  x/1 -> [x]
  [N] -> If/1
  If/1 -> If Action Subsystem/Action
  If/2 -> If Action Subsystem1/Action
  [N] -> If Action Subsystem1/2(N)
  [x] -> If Action Subsystem1/1(x)
  [x] -> If Action Subsystem/1(x)
  If Action Subsystem/1(polyval) -> Merge/1
  If Action Subsystem1/1(polval) -> Merge/2
  Merge/1 -> [polyval]
  [polyval] -> Delay Line/1
  Delay Line/1 -> Frame Conversion/1
  Reshape/1 -> [polyvals]
  [polyvals] -> Memory/1
  [polyvals] -> chebyPol/1  "chebyPol"
  Frame Conversion/1 -> Reshape/1
  Memory/1 -> If Action Subsystem/2(polyvals)

== system simQuadrotor/Controller/Disturbance Estimator/getDisturbance/getDhat/adaptiveGain ==
  psi(z) : Inport
  es : Inport  Port=2
  Gain1 : Gain  Gain=-1
  Math Function : Math  Operator=transpose  SaturateOnIntegerOverflow=on
  P : Constant  Value=Ps  VectorParams1D=off
  Product1 : Product  Multiplication=Matrix(*)  RndMeth=Zero
  Product3 : Product  Multiplication=Matrix(*)  RndMeth=Zero
  Wintegrand : Outport
  wires:
  Product1/1 -> Product3/2
  psi(z)/1 -> Product3/1
  Gain1/1 -> Wintegrand/1
  es/1 -> Math Function/1
  Math Function/1 -> Product1/1
  P/1 -> Product1/2
  Product3/1 -> Gain1/1

== system simQuadrotor/Controller/Disturbance Estimator/getDisturbance/getDhat/getW1 ==
  Wint : Inport
  psiz : Inport  Port=2
  Constant : Constant  Value=Wbnd  VectorParams1D=off
  Constant1 : Constant  Value=epsilontheta
  Discrete-Time Integrator : DiscreteIntegrator  IntegratorMethod=Integration: Trapezoidal  InitialCondition=W0  SampleTime=-1  LimitOutput=on  UpperSaturationLimit=Wbnd  LowerSaturationLimit=-Wbnd
  Gain : Gain  Gain=GammaW
  Math Function : Math  Operator=transpose  SaturateOnIntegerOverflow=on
  Memory4 : Memory  X0=W0  InheritSampleTime=on  LinearizeMemory=on  LinearizeAsDelay=on
  Product : Product  Multiplication=Matrix(*)  RndMeth=Zero
  Projection : Subsystem  TreatAsAtomicUnit=on
  W : Outport
  WTpsi : Outport  Port=2
  wires:
  [WTpsi] -> WTpsi/1
  [Wint] -> Projection/2(y)
  Math Function/1 -> Product/1
  [psiz] -> Product/2
  Discrete-Time Integrator/1 -> Math Function/1, [W], Memory4/1
  Gain/1 -> Discrete-Time Integrator/1
  Projection/1(Proj) -> Gain/1  "WintProj"
  Memory4/1 -> Projection/1(theta)
  Constant/1 -> Projection/3(Thetamax)
  Constant1/1 -> Projection/4(epsilontheta)
  [W] -> W/1
  Wint/1 -> [Wint]
  psiz/1 -> [psiz]
  Product/1 -> [WTpsi]  "WTpsi"

== system simQuadrotor/Controller/Disturbance Estimator/getDisturbance/getDhat/getW2 ==
  Wint : Inport
  psiz : Inport  Port=2
  Constant : Constant  Value=Wbnd  VectorParams1D=off
  Constant1 : Constant  Value=epsilontheta
  Discrete-Time Integrator : DiscreteIntegrator  IntegratorMethod=Integration: Trapezoidal  InitialCondition=W0  SampleTime=-1  LimitOutput=on  UpperSaturationLimit=Wbnd  LowerSaturationLimit=-Wbnd
  Gain : Gain  Gain=GammaW
  Math Function : Math  Operator=transpose  SaturateOnIntegerOverflow=on
  Memory4 : Memory  X0=W0  InheritSampleTime=on  LinearizeMemory=on  LinearizeAsDelay=on
  Product : Product  Multiplication=Matrix(*)  RndMeth=Zero
  Projection : Subsystem  TreatAsAtomicUnit=on
  W : Outport
  WTpsi : Outport  Port=2
  wires:
  Product/1 -> [WTpsi]  "WTpsi"
  psiz/1 -> [psiz]
  Wint/1 -> [Wint]
  [W] -> W/1
  Constant1/1 -> Projection/4(epsilontheta)
  Constant/1 -> Projection/3(Thetamax)
  Memory4/1 -> Projection/1(theta)
  Projection/1(Proj) -> Gain/1  "WintProj"
  Gain/1 -> Discrete-Time Integrator/1
  Discrete-Time Integrator/1 -> Memory4/1, [W], Math Function/1
  [psiz] -> Product/2
  Math Function/1 -> Product/1
  [Wint] -> Projection/2(y)
  [WTpsi] -> WTpsi/1

== system simQuadrotor/Controller/Disturbance Estimator/getDisturbance/getDhat/getW3 ==
  Wint : Inport
  psiz : Inport  Port=2
  Constant : Constant  Value=Wbnd  VectorParams1D=off
  Constant1 : Constant  Value=epsilontheta
  Discrete-Time Integrator : DiscreteIntegrator  IntegratorMethod=Integration: Trapezoidal  InitialCondition=W0  SampleTime=-1  LimitOutput=on  UpperSaturationLimit=Wbnd  LowerSaturationLimit=-Wbnd
  Gain : Gain  Gain=GammaW
  Math Function : Math  Operator=transpose  SaturateOnIntegerOverflow=on
  Memory4 : Memory  X0=W0  InheritSampleTime=on  LinearizeMemory=on  LinearizeAsDelay=on
  Product : Product  Multiplication=Matrix(*)  RndMeth=Zero
  Projection : Subsystem  TreatAsAtomicUnit=on
  W : Outport
  WTpsi : Outport  Port=2
  wires:
  [WTpsi] -> WTpsi/1
  [Wint] -> Projection/2(y)
  Math Function/1 -> Product/1
  [psiz] -> Product/2
  Discrete-Time Integrator/1 -> Math Function/1, [W], Memory4/1
  Gain/1 -> Discrete-Time Integrator/1
  Projection/1(Proj) -> Gain/1  "WintProj"
  Memory4/1 -> Projection/1(theta)
  Constant/1 -> Projection/3(Thetamax)
  Constant1/1 -> Projection/4(epsilontheta)
  [W] -> W/1
  Wint/1 -> [Wint]
  psiz/1 -> [psiz]
  Product/1 -> [WTpsi]  "WTpsi"
